simulink model "quadcop"  (R2025b)
settings: Solver=ode4  StartTime=0.0  StopTime=30  FixedStep=Ts_inner  RelTol=1e-3
InitFcn:
  | xi0  = [quadcop.x0; quadcop.v0];        % Luenberger-Init: Position = erster Mocap-Wert, v=0
undefined symbols (not defined in the file): Ts_gcs
libraries: sldrtlib x1
settings Model: DataDictionary=project.sldd  Creator=Nick  LastModifiedBy=Rakete
settings SolverCC: AutoInsertRateTranBlk=on

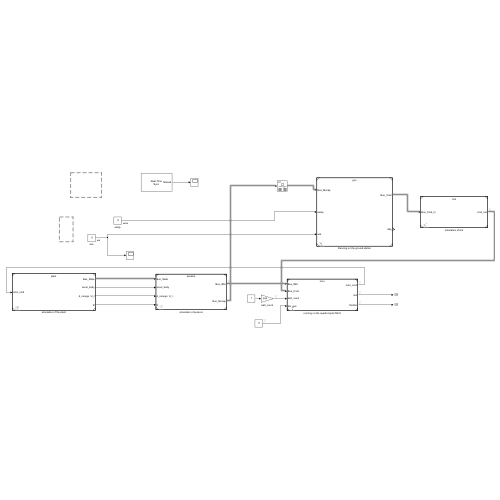
[thumbnail: Simulink's stored preview of the top-level diagram]
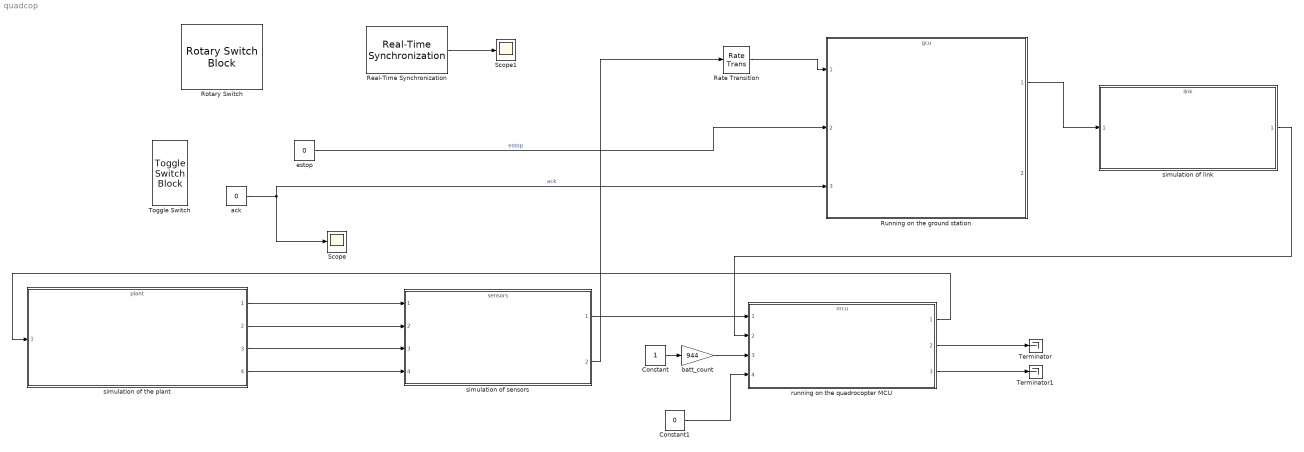
== system quadcop ==
  Constant : Constant
  Constant1 : Constant  Value=0  OutDataTypeStr=boolean
  Rate Transition : RateTransition  OutPortSampleTime=Ts_gcs
  Real-Time Synchronization : sldrtlib/Real-Time Synchronization  SampleTime=Ts_gcs  MaxMissedTicks=inf  ShowMissedTicks=on  YieldWhenWaiting=off
  Rotary Switch : RotarySwitchBlock
  Running on the ground station : ModelReference  ModelNameDialog=gcu.slx  UsingDefaultArgumentValue=0,0,0  SimulationMode=Normal  ModelReferenceVersion=1.334
  Scope : Scope
      settings: ActiveDisplayYMinimum=-0.12499999999999997  ActiveDisplayYMaximum=1.125
  Scope1 : Scope
      settings: ActiveDisplayYMinimum=-248.37499999999994  ActiveDisplayYMaximum=2235.375
  Terminator : Terminator
  Terminator1 : Terminator
  Toggle Switch : ToggleSwitchBlock
  ack : Constant  Value=0  OutDataTypeStr=boolean
  batt_count : Gain  Gain=944
  estop : Constant  Value=0  OutDataTypeStr=uint8
  running on the quadrocopter MCU : ModelReference  ModelNameDialog=mcu.slx  SimulationMode=Normal  ModelReferenceVersion=1.315
  simulation of link : ModelReference  ModelNameDialog=link.slx  SimulationMode=Normal  ModelReferenceVersion=1.137
  simulation of sensors : ModelReference  ModelNameDialog=sensors.slx  SimulationMode=Normal  ModelReferenceVersion=1.89
  simulation of the plant : ModelReference  ModelNameDialog=plant.slx  SimulationMode=Normal  ModelReferenceVersion=1.211
  wires:
  simulation of the plant/1 -> simulation of sensors/1
  simulation of the plant/2 -> simulation of sensors/2
  simulation of the plant/3 -> simulation of sensors/3
  simulation of the plant/4 -> simulation of sensors/4
  simulation of sensors/1 -> running on the quadrocopter MCU/1
  simulation of sensors/2 -> Rate Transition/1
  Running on the ground station/1 -> simulation of link/1
  Rate Transition/1 -> Running on the ground station/1
  simulation of link/1 -> running on the quadrocopter MCU/2
  Real-Time Synchronization/1 -> Scope1/1
  ack/1 -> Running on the ground station/3, Scope/1  "ack"
  Constant/1 -> batt_count/1
  batt_count/1 -> running on the quadrocopter MCU/3
  running on the quadrocopter MCU/1 -> simulation of the plant/1
  running on the quadrocopter MCU/2 -> Terminator/1
  running on the quadrocopter MCU/3 -> Terminator1/1
  Constant1/1 -> running on the quadrocopter MCU/4
  estop/1 -> Running on the ground station/2  "estop"
